simulink model "target_cam_robot_demo"  (Simulink 7.3)
settings: Solver=FixedStepDiscrete  SolverMode=SingleTasking  StartTime=0.0  StopTime=inf  RelTol=1e-3
PreLoadFcn:
  | waijung.modelPreload; % Required for working with Waijung Blockset. Do not remove.
undefined symbols (not defined in the file): A1, A2, A7, B10, B11, B12, C1, C2, C3, C4, C5, G14, H2, H3, H6, H7, HSEOSC, Link, LQFP176, ST, STM32F417IG
libraries: simulink x12, stm32f4_i2c_lib x8, stm32f4_tim_lib x2, stm32f4_io_lib x2, waijung_webserver x2, waijung_socket_lib x2, stm32f4_rcc_lib x1, stm32f4_device_config_lib x1, waijung_addon_module x1
(part 1 of 2)
CloseFcn:
  | waijung.modelClose; % Required for working with Waijung Blockset. Do not remove.
settings Model: Creator=Krisada  LastModifiedBy=Krisada
settings OptimizationCC: OptimizeModelRefInitCode=on  LifeSpan=1
settings HardwareCC: ProdEndianess=LittleEndian  ProdHWDeviceType=ARM Compatible->Cortex - M4  TargetEndianess=LittleEndian  TargetHWDeviceType=ARM Compatible->Cortex - M4
settings RTWCC: SystemTargetFile=stm32f4.tlc  GenerateMakefile=off  TemplateMakefile=ert_default_tmf  Description=STM32F4 Target  ProcessScript=stm32f4_make_rtw_hook
settings CodeAppCC: IgnoreCustomStorageClasses=off
settings STFCustomTargetCC: ModelReferenceCompliant=off  CombineOutputUpdateFcns=on  ERTCustomFileBanners=on  SupportContinuousTime=off  SupportNonInlinedSFcns=off  SystemTargetFile=stm32f4.tlc
settings ERTTargetCC: MultiwordLength=2048  ModelReferenceCompliant=off  ParMdlRefBuildCompliant=off  CompOptLevelCompliant=off  ERTFirstTimeCompliant=off  ModelStepFunctionPrototypeControlCompliant=off  CPPClassGenCompliant=off  ExtModeMexFile=noextcomm  InlinedParameterPlacement=NonHierarchical  ERTSrcFileBannerTemplate=stm32f4_code_template.cgt  ERTHdrFileBannerTemplate=stm32f4_code_template.cgt  ERTDataSrcFileTemplate=stm32f4_code_template.cgt  ERTDataHdrFileTemplate=stm32f4_code_template.cgt  ERTCustomFileTemplate=stm32f4_file_process.tlc

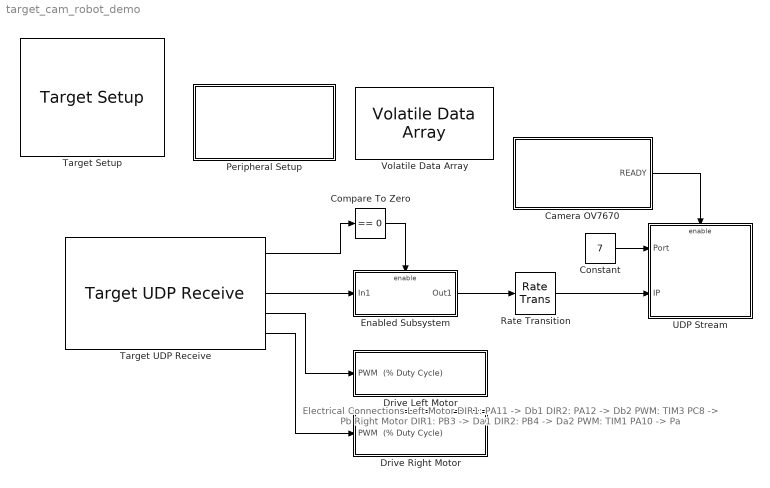
== system target_cam_robot_demo ==
  note: Electrical Connections
      |
      | Left Motor
      | DIR1: PA11 -> Db1
      | DIR2: PA12 ->  Db2
      | PWM: TIM3 PC8 -> Pb
      |
      | Right Motor
      | DIR1: PB3 -> Da1
      | DIR2: PB4 ->  Da2
      | PWM: TIM1 PA10 -> Pa
  Camera OV7670 : Subsystem  mask{camera=OV7670, storagename=ExtRAM, xclkfreq=8MHz(MCO), imgsize=120 x 160, module=1, slvaddr=hex2dec('42'), sampletime=0.01}
      mask prompts: storagename "Output buffer"; xclkfreq "XCLK input frequency"; imgsize "Image size"; module "I2C Module"; slvaddr "I2C Slave address"; sampletime "Sample time (sec)"
      mask init:
      | waijung_image_sensor_callback('init');
      mask StyleString: popup(OV7670),popup(Output|ExtRAM),popup(8MHz(MCO)|24MHz),popup(120 x 160|240 x 320|480 x 640),popup(1|2|3),edit,edit
      mask CallbackString: waijung_image_sensor_callback('camera');|waijung_image_sensor_callback('storagename');|||waijung_image_sensor_callback('module');||
      mask Display: text(0.5, 0.5, '[OV7670]\nPort: I2C1','ver','middle','hor','center');port_label('output', 1,'READY');
  Compare To Zero : simulink/Logic and Bit Operations/Compare To Zero  SystemSampleTime=-1  relop===  LogicOutDataTypeMode=uint8  ZeroCross=off
  Constant : Constant  Value=7  OutDataTypeMode=uint16  OutDataType=fixdt(1, 16)  OutScaling=2^0  OutDataTypeStr=uint16
  Drive Left Motor : Subsystem
  Drive Right Motor : Subsystem
  Enabled Subsystem : Subsystem  TreatAsAtomicUnit=on
  Peripheral Setup : Subsystem
  Rate Transition : RateTransition
  Target Setup : stm32f4_device_config_lib/Target Setup  Priority=100  compiler=GNU ARM  previous_compiler=GNU ARM  mcu=STM32F417IG (LQFP176)  mcustr=STM32F417IG  clockconfig=HSEOSC-8MHz  system_stm32f4xx_c_path=F:\trunk\targets\stm32f4_target\stm32f4\utils\system_stm32f4xx_default\STM32F40_41xxx\hseosc8mhz  showmemoryconfiguration=off  stacksize=0x2000  heapsize=0x2000  enableautocompiledownload=on  fullchiperase=off  programmerinterface=ST-Link  editctrlstr=on  compilercontrolstr=$(patsubst %, -I%, .) -mcpu=cortex-m4 -mthumb -mthumb-interwork -mfloat-abi=hard -mfpu=fpv4-sp-d16 -ffast-math -Wall -Wextra -Ofast  assemblercontrolstr=$(patsubst %, -I%, .) -mcpu=cortex-m4 -mthumb -mthumb-interwork -mfloat-abi=hard -mfpu=fpv4-sp-d16 -ffast-math -Wall -Wextra -Ofast -Wa,-amhls=$(<:.s=.lst) -D__STACK_SIZE=$(STACK_SIZE) -D__HEAP_SIZE=$(HEAP_SIZE)  linkercontrolstr=-T$(LD_SCRIPT) -g -Wl,-Map=$(MAP),--cref,--no-warn-mismatch -mcpu=cortex-m4 -mthumb -mthumb-interwork -mfloat-abi=hard -mfpu=fpv4-sp-d16 -specs=nosys.specs  runafterdownload=on  execprofile=None  profileruart=3  profilerbaud=500000  profilertxpin=D8  profilerinitstr=0.0001,168000000,16800,500000,0  manualsetsampletime=off  sampletime=0.0001  blockid=TargetSetup  systickreloadvalue=16800  hseval=8000000  lastprofileruart=3  hclk=168000000  flashorigin=0x08000000  flashlength=0x100000  ramorigin=0x20000000  ramlength=0x20000  useextram=off
  Target UDP Receive : waijung_socket_lib/Target UDP Receive  conf=TargetReceive  protocol=UDP  port=7  address=192.168.1.21  echo=off  transfer=Non-blocking  timeout=5  datasource=Ports  datatype=uint8  datacount=2  porttype_double=2  porttype_single=0  porttype_int8=0  porttype_uint8=0  porttype_int16=0  porttype_uint16=0  porttype_int32=0  porttype_uint32=0  portpinstr=0  sampletime=inf  blockid=TargetUDPReceive  inputporttype=[]  inputportwidth=[]  inputportlabel={}  outputporttype=[7,5,3,0,0]  outputportwidth=[1,1,4,]  outputportlabel={'Status','Remote Port','Remote IP(1:4)','double D0','double D1'}  compat=0  optionstring="[\"UDP\",\"7\",\"192\",\"168\",\"1\",\"21\",\"Non-blocking\",\"PortData\",\"uint8_t\",\"2\",\"Receive\",\"off\",\"\",\"\",\"\",\"\",\"\",\"\",\"\"]"  options=[7,2,1,5000,0]
  UDP Stream : Subsystem  TreatAsAtomicUnit=on
  Volatile Data Array : waijung_addon_module/Data Storage/Volatile Data Array  conf=Setup  specificaddress=off  storagename=Output  memoryaddress=hex2dec('64000000')  storagetype=uint16  datasize=160*120  varname=VolatileDataArray_Output  datatype=double  datacount=0  portpinstr=0  sampletime=inf  blockid=VolatileDataArray  inputporttype=[]  inputportwidth=[]  inputportlabel={}  outputporttype=[]  outputportwidth=[]  outputportlabel={}  compat=0  optionstring="[\"off\",\"?\",\"Output\",\"uint16\",\"19200\",\"VolatileDataArray_Output\",\"uint16_t\",\"Param1\"]"
  wires:
  Constant/1 -> UDP Stream/1(Port)
  Target UDP Receive/3 -> Enabled Subsystem/1(In1)
  Enabled Subsystem/1(Out1) -> Rate Transition/1
  Target UDP Receive/1 -> Compare To Zero/1
  Compare To Zero/1 -> Enabled Subsystem/Enable
  Camera OV7670/1(READY) -> UDP Stream/Enable
  Rate Transition/1 -> UDP Stream/2(IP)
  Target UDP Receive/4 -> Drive Left Motor/1(PWM  (% Duty Cycle))
  Target UDP Receive/5 -> Drive Right Motor/1(PWM  (% Duty Cycle))

== system target_cam_robot_demo/Camera OV7670 ==
  Capture_ : Subsystem  TreatAsAtomicUnit=on
  Init_ : Subsystem
  Logical Operator : Logic  Operator=NOT  AllPortsSameDT=off  OutDataTypeMode=boolean  LogicDataType=fixdt(0, 8)  OutDataTypeStr=boolean
  Memory : Memory  InheritSampleTime=on
  Rate Transition : RateTransition  OutPortSampleTime=sampletime
  READY : Outport  OutDataType=fixdt(1, 16)  OutScaling=2^0
  wires:
  Rate Transition/1 -> Capture_/Enable
  Logical Operator/1 -> Init_/Enable
  Memory/1 -> Rate Transition/1, Logical Operator/1
  Init_/1(Out1) -> Memory/1
  Capture_/1(SUCCESS) -> READY/1

== system target_cam_robot_demo/Drive Left Motor ==
  PWM  (% Duty Cycle) : Inport
  Abs : Abs  OutDataType=fixdt(1, 16)  OutScaling=2^0
  Basic PWM : S-Function  FunctionName=stm32f4_basicpwm  Parameters=timer,pwmperiod,ch1pin,ch2pin,ch3pin,ch4pin,sampletime,sampletimestr,blockid,apb,portstr,pinstr,pinmat,timarr,timprescale,chmat,polaritystr  EnableBusSupport=off  mask(stm32f4_basicpwm){timer=3, pwmperiod=0.005, polarity=Active High, polaritystr=TIM_OCPolarity_High, ch1pin=Not available - Do not use, ch2pin=Not available - Do not use, ch3pin=C8, ch4pin=Not available - Do not use, sampletime=-1, sampletimestr=0.0001, blockid=DriveLeftMotorBasicPWM, portpinstr=,,C8,, enablecustomportlabel=off, cinputportlabel=In1, In2, In3, In4, coutputportlabel=0, apb=1, portstr=["C"], pinstr=["GPIO_Pin_8"], pinmat=[1 8], timarr=59999, timprescale=6, chmat=[3]}
      mask prompts: pwmperiod "PWM Period (seconds)"; ch1pin "Channel 1"; ch2pin "Channel 2"; ch3pin "Channel 3"; ch4pin "Channel 4"; sampletime "Sample time (sec)"; sampletimestr "Compiled sample time (sec) in string"; portpinstr "Port pin string"; enablecustomportlabel "Enable custom port labels"; cinputportlabel "Custom input port labels (Ex. In1, In2, In3)"; coutputportlabel "Custom output port labels (Ex. Out1, Out2, Out3)"; portstr "Port string"; pinstr "Pin string"; pinmat "Pin matrix"; timarr "Timer ARR"; timprescale "Timer PRESCALE"; chmat "Channel order"
      mask help:
      | This block implements basic Edge-aligned Pulse Width Modulation (PWM) generation.
      | All timers are 16-bit. The PWM period is fixed (per timer).
      mask init:
      | stm32f4_basicpwm_callback('init');
      mask Help: web(fullfile(waijungdocroot,'stm32f4_basicpwm.htm'),'-browser')
      mask StyleString: popup(1|2|3|4|5|8|9|10|11|12|13|14),edit,popup(Active High|Active Low),edit,popup(Not available - Do not use|A6|C6|B4),popup(Not available - Do not use|A7|C7|B5),popup(Not available - Do not use|B0|C8),popup(Not available - Do not use|B1|C9),edit,edit,edit,edit,checkbox,edit,edit,edit,edit,edit,edit,edit,edit,edit
      mask CallbackString: stm32f4_basicpwm_callback('timer');|stm32f4_basicpwm_callback('pwmperiod');|stm32f4_basicpwm_callback('polarity');||stm32f4_basicpwm_callback('ch1pin');|stm32f4_basicpwm_callback('ch2pin');|stm32f4_basicpwm_callback('ch3pin');|stm32f4_basicpwm_callback('ch4pin');|stm32f4_basicpwm_callback('sampletime');|stm32f4_basicpwm_callback('sampletimestr');|stm32f4_basicpwm_callback('blockid');||stm32f4_basicpwm_callback('enablecustomportlabel');|||||||||
      mask Display: text(0.95, 0.5, 'Timer: 3\nPolarity: Active High\nPeriod (sec) 0.005\nTs (sec): 0.0001','ver','middle','hor','right');port_label('input', 1,'CH3 (C8)')
  CCW : Subsystem  TreatAsAtomicUnit=on
  CW : Subsystem  TreatAsAtomicUnit=on
  Demux : Demux  Outputs=2
  Digital Output : stm32f4_io_lib/Digital Output  use_bitband=on  port=A  speed=100  porttype=Open Drain  porttypestr=OD  use_pin0=off  use_pin1=off  use_pin2=off  use_pin3=off  use_pin4=off  use_pin5=off  use_pin6=off  use_pin7=off  use_pin8=off  use_pin9=off  use_pin10=off  use_pin11=on  use_pin12=on  use_pin13=off  use_pin14=off  use_pin15=off  pinstr=GPIO_Pin_11 | GPIO_Pin_12  usedpinarray="[0  0  0  0  0  0  0  0  0  0  0  1  1  0  0  0]"  bitbandingstr=|  sampletime=-1  sampletimestr=0.0001  blockid=DriveLeftMotorDigitalOutput  enablecustomportlabel=off  globalinit=off  cinputportlabel=In1, In2  coutputportlabel=0
      | #define DriveLeftMotorDigitalOutput_A11 Peripheral_BB(GPIOA->ODR, 11)  /* Output pin */
      | #define DriveLeftMotorDigitalOutput_A12 Peripheral_BB(GPIOA->ODR, 12)  /* Output pin */
  If : If  ElseIfExpressions=u1<0
  Merge : Merge  Inputs=3  InitialOutput=[0 0]
  STOP : Subsystem  TreatAsAtomicUnit=on
  wires:
  Abs/1 -> Basic PWM/1
  If/1 -> CW/Action
  If/2 -> CCW/Action
  If/3 -> STOP/Action
  CW/1(DIR) -> Merge/1
  CCW/1(DIR) -> Merge/2
  STOP/1(DIR) -> Merge/3
  Merge/1 -> Demux/1
  Demux/1 -> Digital Output/1
  PWM  (% Duty Cycle)/1 -> Abs/1, If/1
  Demux/2 -> Digital Output/2

== system target_cam_robot_demo/Drive Right Motor ==
  PWM  (% Duty Cycle) : Inport
  Abs : Abs  OutDataType=fixdt(1, 16)  OutScaling=2^0
  Basic PWM : S-Function  FunctionName=stm32f4_basicpwm  Parameters=timer,pwmperiod,ch1pin,ch2pin,ch3pin,ch4pin,sampletime,sampletimestr,blockid,apb,portstr,pinstr,pinmat,timarr,timprescale,chmat,polaritystr  EnableBusSupport=off  mask(stm32f4_basicpwm){timer=1, pwmperiod=0.005, polarity=Active High, polaritystr=TIM_OCPolarity_High, ch1pin=Not available - Do not use, ch2pin=Not available - Do not use, ch3pin=A10, ch4pin=Not available - Do not use, sampletime=-1, sampletimestr=0.0001, blockid=DriveRightMotorBasicPWM, portpinstr=,,A10,, enablecustomportlabel=off, cinputportlabel=In1, In2, In3, In4, coutputportlabel=0, apb=2, portstr=["A"], pinstr=["GPIO_Pin_10"], pinmat=[1 10], timarr=64614, timprescale=12, chmat=[3]}
      mask prompts: pwmperiod "PWM Period (seconds)"; ch1pin "Channel 1"; ch2pin "Channel 2"; ch3pin "Channel 3"; ch4pin "Channel 4"; sampletime "Sample time (sec)"; sampletimestr "Compiled sample time (sec) in string"; portpinstr "Port pin string"; enablecustomportlabel "Enable custom port labels"; cinputportlabel "Custom input port labels (Ex. In1, In2, In3)"; coutputportlabel "Custom output port labels (Ex. Out1, Out2, Out3)"; portstr "Port string"; pinstr "Pin string"; pinmat "Pin matrix"; timarr "Timer ARR"; timprescale "Timer PRESCALE"; chmat "Channel order"
      mask help:
      | This block implements basic Edge-aligned Pulse Width Modulation (PWM) generation.
      | All timers are 16-bit. The PWM period is fixed (per timer).
      mask init:
      | stm32f4_basicpwm_callback('init');
      mask Help: web(fullfile(waijungdocroot,'stm32f4_basicpwm.htm'),'-browser')
      mask StyleString: popup(1|2|3|4|5|8|9|10|11|12|13|14),edit,popup(Active High|Active Low),edit,popup(Not available - Do not use|E9|A8),popup(Not available - Do not use|E11|A9),popup(Not available - Do not use|E13|A10),popup(Not available - Do not use|E14|A11),edit,edit,edit,edit,checkbox,edit,edit,edit,edit,edit,edit,edit,edit,edit
      mask CallbackString: stm32f4_basicpwm_callback('timer');|stm32f4_basicpwm_callback('pwmperiod');|stm32f4_basicpwm_callback('polarity');||stm32f4_basicpwm_callback('ch1pin');|stm32f4_basicpwm_callback('ch2pin');|stm32f4_basicpwm_callback('ch3pin');|stm32f4_basicpwm_callback('ch4pin');|stm32f4_basicpwm_callback('sampletime');|stm32f4_basicpwm_callback('sampletimestr');|stm32f4_basicpwm_callback('blockid');||stm32f4_basicpwm_callback('enablecustomportlabel');|||||||||
      mask Display: text(0.95, 0.5, 'Timer: 1\nPolarity: Active High\nPeriod (sec) 0.005\nTs (sec): 0.0001','ver','middle','hor','right');port_label('input', 1,'CH3 (A10)')
  CCW : Subsystem  TreatAsAtomicUnit=on
  CW : Subsystem  TreatAsAtomicUnit=on
  Demux : Demux  Outputs=2
  Digital Output : stm32f4_io_lib/Digital Output  use_bitband=on  port=B  speed=100  porttype=Open Drain  porttypestr=OD  use_pin0=off  use_pin1=off  use_pin2=off  use_pin3=on  use_pin4=on  use_pin5=off  use_pin6=off  use_pin7=off  use_pin8=off  use_pin9=off  use_pin10=off  use_pin11=off  use_pin12=off  use_pin13=off  use_pin14=off  use_pin15=off  pinstr=GPIO_Pin_3 | GPIO_Pin_4  usedpinarray="[0  0  0  1  1  0  0  0  0  0  0  0  0  0  0  0]"  bitbandingstr=|  sampletime=-1  sampletimestr=0.0001  blockid=DriveRightMotorDigitalOutput  enablecustomportlabel=off  globalinit=off  cinputportlabel=In1, In2  coutputportlabel=0
      | #define DriveRightMotorDigitalOutput_B3 Peripheral_BB(GPIOB->ODR, 3)  /* Output pin */
      | #define DriveRightMotorDigitalOutput_B4 Peripheral_BB(GPIOB->ODR, 4)  /* Output pin */
  If : If  ElseIfExpressions=u1<0
  Merge : Merge  Inputs=3  InitialOutput=[0 0]
  STOP : Subsystem  TreatAsAtomicUnit=on
  wires:
  PWM  (% Duty Cycle)/1 -> If/1, Abs/1
  Demux/2 -> Digital Output/2
  Demux/1 -> Digital Output/1
  Merge/1 -> Demux/1
  STOP/1(DIR) -> Merge/3
  CCW/1(DIR) -> Merge/2
  CW/1(DIR) -> Merge/1
  If/3 -> STOP/Action
  If/2 -> CCW/Action
  If/1 -> CW/Action
  Abs/1 -> Basic PWM/1

== system target_cam_robot_demo/Enabled Subsystem ==
  In1 : Inport  OutDataType=fixdt(1, 16)  OutScaling=2^0
  Enable : EnablePort
  Out1 : Outport  OutDataType=fixdt(1, 16)  OutScaling=2^0  InitialOutput=[192 168 1 48]
  wires:
  In1/1 -> Out1/1

== system target_cam_robot_demo/Peripheral Setup ==
  Ethernet Application Setup : waijung_webserver/Ethernet Application Setup  conf=Setup  ipaddress=192.168.1.31  netmask=255.255.255.0  gateway=192.168.1.1  macaddress=02-00-00-00-00-00  dhcp=off  timerscaler=100  portpinstr=0  sampletime=0.0001  blockid=PeripheralSetupEthernetApplicationSetup  inputporttype=[]  inputportwidth=[]  inputportlabel={}  outputporttype=[]  outputportwidth=[]  outputportlabel={}  compat=0  optionstring="[\"Dummy\",\"192\",\"168\",\"1\",\"31\",\"255\",\"255\",\"255\",\"0\",\"192\",\"168\",\"1\",\"1\",\"02\",\"00\",\"00\",\"00\",\"00\",\"00\",\"off\",\"100\"]"
  Ethernet Link Setup : waijung_webserver/Ethernet Link Setup  conf=Setup  interfacepin=Profile #2  wj_interfacetype=MII  pin_mdio=A2  pin_mdc=C1  pin_pps=Not used  pin_crs=H2  pin_col=H3  pin_dv=A7  pin_rxclk=A1  pin_rxer=B10  pin_rxd0=C4  pin_rxd1=C5  pin_rxd2=H6  pin_rxd3=H7  pin_txclk=C3  pin_txen=B11  pin_txd0=B12  pin_txd1=G14  pin_txd2=C2  pin_txd3=E2  portpinstr=H2,A1,A2,H3,A7,H6,H7,E2,B10,B11,B12,G14,C1,C2,C3,C4,C5  sampletime=inf  blockid=PeripheralSetupEthernetLinkSetup  inputporttype=[]  inputportwidth=[]  inputportlabel={}  outputporttype=[]  outputportwidth=[]  outputportlabel={}  compat=0  optionstring="[\"xxx\",\"on\",\"on\",\"on\",\"off\",\"on\",\"off\",\"on\",\"on\",\"off\",\"on\",\"on\",\"on\",\"on\",\"on\",\"on\",\"on\",\"off\",\"on\",\"on\",\"on\",\"on\",\"on\",\"on\",\"on\",\"on\",\"on\",\"on\",\"H\",\"2\",\"A\",\"1\",\"A\",\"2\",\"H\",\"3\",\"A\",\"7\",\"H\",\"6\",\"H\",\"7\",\"N\",\"ot used\",\"E\",\"2\",\"B\",\"10\",\"B\",\"11\",\"B\",\"12\",\"G\",\"14\",\"C\",\"1\",\"C\",\"2\",\"C\",\"3\",\"C\",\"4\",\"C\",\"5\",\"MII\"]"
  I2C Master Setup : S-Function  FunctionName=stm32f4_i2c  Parameters=configuration,module,transfer,clkspeed,timeout,sdapin,sclpin,writecount,readcount,inputtypearray,outputtypearray,confstr,sampletime,sampletimestr,blockid  EnableBusSupport=off  mask(stm32f4_i2c){configuration=Setup, module=1, lastmodule=1, transfer=Blocking, dutycycle=TLow/THigh = 2, clkspeed=100, timeout=25, writecount=0, readcount=0, sdapin=B7, sclpin=B6, waitwritetime=0, inputtypearray=[0], outputtypearray=[0], confstr=["B","7","B","6","1","1","6","0","I2C_DutyCycle_2","0","off"], sampletime=-1, sampletimestr=0.0001, blockid=PeripheralSetupI2CMasterSetup}
      mask prompts: module "I2C Module"; lastmodule "Last module"; transfer "Transfer mode"; dutycycle "Duty cycle in fast mode"; clkspeed "Clock speed (kHz)"; timeout "Timeout (ms)"; writecount "Bytes write count"; readcount "Bytes read count"; sdapin "SDA pin"; sclpin "SCL pin"; waitwritetime "Wait write time (ms), default is 0"; inputtypearray "Input type array"; outputtypearray "Output type array"; confstr "Configuration string"; sampletime "Sample time (sec)"; sampletimestr "Compiled sample time (sec) in string"
      mask init:
      | stm32f4_i2c_callback('init');
      mask Help: web(fullfile(waijungdocroot,'stm32f4_i2c_setup.htm'), '-browser')
      mask StyleString: popup(Setup|Transaction),popup(1|2|3),edit,popup(Blocking|Non-blocking),popup(TLow/THigh = 16/9|TLow/THigh = 2),edit,edit,edit,edit,popup(Not used|B7|B9),popup(Not used|B6|B8),edit,edit,edit,edit,edit,edit,edit
      mask CallbackString: stm32f4_i2c_callback('configuration');|stm32f4_i2c_callback('module');|||stm32f4_i2c_callback('dutycycle');|||stm32f4_i2c_callback('writecount');|stm32f4_i2c_callback('readcount');|stm32f4_i2c_callback('sdapin');|stm32f4_i2c_callback('sclpin');||||stm32f4_i2c_callback('confstr');|stm32f4_i2c_callback('sampletime');|stm32f4_i2c_callback('sampletimestr');|stm32f4_i2c_callback('blockid');
      mask Display: text(0.5, 0.5, 'Module: I2C1\nClock: 100kHz\nSDA/SCL Pin: B7/B6','ver','middle','hor','center');
  MCO : stm32f4_rcc_lib/MCO  conf=MCO  module=1  source=HSE  div=Div_1  sampletime=inf  sampletimestr=0.0001  blockid=PeripheralSetupMCO  inputarray=[]  inputlabelarray={}  outputarray=[]  outputlabelarray={}  compat=0  confstr="[\"1\",\"HSE\",\"Div_1\"]"

== system target_cam_robot_demo/UDP Stream ==
  Port : Inport  OutDataType=fixdt(1, 16)  OutScaling=2^0
  IP : Inport  Port=2  OutDataType=fixdt(1, 16)  OutScaling=2^0
  Enable : EnablePort
  Target UDP Send : waijung_socket_lib/Target UDP Send  conf=TargetSend  protocol=UDP  variableipport=on  port=7  address=192.168.1.33  echo=off  transfer=Non-blocking  timeout=5  datasource=BufferStream  streamsource=Output  streamsize=1024  datatype=uint16  datacount=120*160  porttype_double=0  porttype_single=0  porttype_int8=0  porttype_uint8=0  porttype_int16=0  porttype_uint16=0  porttype_int32=0  porttype_uint32=1  portpinstr=0  sampletime=-1  blockid=UDPStreamTargetUDPSend  inputporttype=[5,3,]  inputportwidth=[1,4,]  inputportlabel={'Port','IP',}  outputporttype=[7]  outputportwidth=[]  outputportlabel={'Status'}  compat=0  optionstring="[\"UDP\",\"7\",\"192\",\"168\",\"1\",\"33\",\"Non-blocking\",\"BufferStream\",\"uint16_t\",\"120*160\",\"Send\",\"off\",\"on\",\"Output\",\"VolatileDataArray_Output\",\"uint16\",\"19200\",\"38400\",\"1024\"]"  options=[7,2,0,5000,1]
  Terminator : Terminator
  wires:
  Port/1 -> Target UDP Send/1
  IP/1 -> Target UDP Send/2
  Target UDP Send/1 -> Terminator/1

== system target_cam_robot_demo/Camera OV7670/Capture_ ==
  Enable : EnablePort
  Compare To Zero : simulink/Logic and Bit Operations/Compare To Zero  SystemSampleTime=-1  relop===  LogicOutDataTypeMode=uint8  ZeroCross=off
  DCMI Capture : S-Function  FunctionName=stm32f4_dcmi  Parameters=conf,inputporttype,inputportwidth,outputporttype,outputportwidth,optionstring,sampletime,blockid  EnableBusSupport=off  mask(stm32f4_dcmi){conf=DCMI, capturemode=SnapShot, synchronizemode=Hardware, pclkpolarity=Falling, vspolarity=High, hspolarity=High, capturerate=All, capturesize=120*160*2, storagename=<Manual Configure>, varname=VolatileDataArray_Output, storagetype=uint16, storagesize=120*160, remap=Profile #2, sampletime=inf, blockid=CameraOV7670Capture_DCMICapture, inputporttype=[], inputportwidth=[], inputportlabel={}, outputporttype=[7], outputportwidth=[], outputportlabel={'Status'}, compat=0, optionstring=["DCMI","SnapShot","Hardware","Falling","High","High","All","0","HalfWord","9600","0","0","VolatileDataArray_Output"," "," "," ","1","0","0","0","0","0","0","1","1","A","6","I","5","H","8","H","9","H","10","H","11","H","12","H","14","I","4","I","6","I","7"], portpinstr=A6,I5,H8,H9,H10,H11,H12,H14,I4,I6,I7}
      mask prompts: conf "Configuration"; capturemode "Capture mode"; synchronizemode "Synchronization Mode"; pclkpolarity "Pixel clock polarity"; vspolarity "Vertical synchronization polarity"; hspolarity "Horizontal synchronization polarity"; capturerate "Capture rate"; capturesize "Capture data size (Bytes)"; storagename "Output buffer"; varname "Output buffer var name"; storagetype "Output buffer var type"; storagesize "Output buffer size (Total bytes must be equal to, or greater than DMA Transfer size)"; remap "Remap DCMI pins"; sampletime "Sample time (sec)"; inputporttype "Input port"; inputportwidth "Input Port Width"; inputportlabel "Input port label"; outputporttype "Output port"; outputportwidth "Output Port Width"; outputportlabel "Output port label"; compat "Compatibility (Reserved for future use)"; optionstring "Configuration String"; portpinstr "Port Pin String"
      mask help:
      | Synchronize mode:
      |  - Hardware: Hardware synchronization data capture is synchronized with the HSYNC/VSYNC signals.
      |  - Embedded: Embedded synchronization data capture is synchronized with synchronization codes embedded in the data flow.
      | Pixel clock polarity:
      |  - Falling: Pixel clock active on Falling edge.
      |  - Rising: Pixel clock active on Rising edge.
      | Vertical, Horizontal sychronization polarity:
      |  - Low: vertical synchronization active Low.
      |  - High: Vertical synchronization active High.
      | Capture rate:
      |  - All: All frames are captured.
      |  - 1of2: Every alternate frame captured.
      |  - 1of4: On frame in 4 frames captured.
      | Pins Profile:
      | Set of configuration pins for: PIXCLK, VSYNC, HSYNC, D0, D1, .., D7 corresponding.
      |  - Profile #1: PA6, PB7, PA4, PC6, PC7,  PE0,  PE1,  PE4,  PB6, PE5, PE6
      |  - Profile #2: PA6, PI5, PH8, PH9, PH10, PH11, PH12, PH14, PI4, PI6, PI7
      mask init:
      | stm32f4_dcmi_callback('init');
      mask Help: web(fullfile(waijungdocroot,'stm32f4_dcmi.htm'), '-browser')
      mask StyleString: popup(DCMI),popup(Continuous|SnapShot),popup(Hardware|Embedded),popup(Falling|Rising),popup(High|Low),popup(High|Low),popup(All|1of2|1of4),edit,popup(<Manual Configure>),edit,popup(double|single|int8|uint8|int16|uint16|int32|uint32),edit,popup(Profile #1|Profile #2),edit,edit,edit,edit,edit,edit,edit,edit,edit,edit,edit
      mask CallbackString: stm32f4_dcmi_callback('conf');||||||||stm32f4_dcmi_callback('storagename');|||stm32f4_dcmi_callback('storagesize');|stm32f4_dcmi_callback('remap');|stm32f4_dcmi_callback('sampletime');|stm32f4_dcmi_callback('blockid');|||||||||
      mask Display: text(0.05, 0.5, 'Size: 38400\nPins: Profile #2\nTs (sec): 0.01','ver','middle','hor','left'); port_label('output', 1,'Status');
  SUCCESS : Outport  OutDataType=fixdt(1, 16)  OutScaling=2^0
  wires:
  DCMI Capture/1 -> Compare To Zero/1
  Compare To Zero/1 -> SUCCESS/1

== system target_cam_robot_demo/Camera OV7670/Init_ ==
  Enable : EnablePort
  While Iterator_ : Subsystem  TreatAsAtomicUnit=on
  Out1 : Outport
  wires:
  While Iterator_/1(Ready) -> Out1/1

== system target_cam_robot_demo/Drive Left Motor/CCW ==
  Action Port : ActionPort  ActionType=elseif
  Constant : Constant  Value=0  OutDataType=fixdt(1, 16)  OutScaling=2^0
  Constant1 : Constant  OutDataType=fixdt(1, 16)  OutScaling=2^0
  Mux : Mux  Inputs=2
  DIR : Outport  OutDataType=fixdt(1, 16)  OutScaling=2^0  InitialOutput=[0 0]
  wires:
  Mux/1 -> DIR/1
  Constant1/1 -> Mux/2
  Constant/1 -> Mux/1

== system target_cam_robot_demo/Drive Left Motor/CW ==
  Action Port : ActionPort  ActionType=then
  Constant : Constant  OutDataType=fixdt(1, 16)  OutScaling=2^0
  Constant1 : Constant  Value=0  OutDataType=fixdt(1, 16)  OutScaling=2^0
  Mux : Mux  Inputs=2
  DIR : Outport  OutDataType=fixdt(1, 16)  OutScaling=2^0  InitialOutput=[0 0]
  wires:
  Constant/1 -> Mux/1
  Constant1/1 -> Mux/2
  Mux/1 -> DIR/1

== system target_cam_robot_demo/Drive Left Motor/STOP ==
  Action Port : ActionPort  ActionType=else
  Constant : Constant  Value=0  OutDataType=fixdt(1, 16)  OutScaling=2^0
  Constant1 : Constant  Value=0  OutDataType=fixdt(1, 16)  OutScaling=2^0
  Mux : Mux  Inputs=2
  DIR : Outport  OutDataType=fixdt(1, 16)  OutScaling=2^0  InitialOutput=[0 0]
  wires:
  Constant/1 -> Mux/1
  Constant1/1 -> Mux/2
  Mux/1 -> DIR/1

== system target_cam_robot_demo/Drive Right Motor/CCW ==
  Action Port : ActionPort  ActionType=elseif
  Constant : Constant  Value=0  OutDataType=fixdt(1, 16)  OutScaling=2^0
  Constant1 : Constant  OutDataType=fixdt(1, 16)  OutScaling=2^0
  Mux : Mux  Inputs=2
  DIR : Outport  OutDataType=fixdt(1, 16)  OutScaling=2^0  InitialOutput=[0 0]
  wires:
  Constant/1 -> Mux/1
  Constant1/1 -> Mux/2
  Mux/1 -> DIR/1

== system target_cam_robot_demo/Drive Right Motor/CW ==
  Action Port : ActionPort  ActionType=then
  Constant : Constant  OutDataType=fixdt(1, 16)  OutScaling=2^0
  Constant1 : Constant  Value=0  OutDataType=fixdt(1, 16)  OutScaling=2^0
  Mux : Mux  Inputs=2
  DIR : Outport  OutDataType=fixdt(1, 16)  OutScaling=2^0  InitialOutput=[0 0]
  wires:
  Mux/1 -> DIR/1
  Constant1/1 -> Mux/2
  Constant/1 -> Mux/1

== system target_cam_robot_demo/Drive Right Motor/STOP ==
  Action Port : ActionPort  ActionType=else
  Constant : Constant  Value=0  OutDataType=fixdt(1, 16)  OutScaling=2^0
  Constant1 : Constant  Value=0  OutDataType=fixdt(1, 16)  OutScaling=2^0
  Mux : Mux  Inputs=2
  DIR : Outport  OutDataType=fixdt(1, 16)  OutScaling=2^0  InitialOutput=[0 0]
  wires:
  Mux/1 -> DIR/1
  Constant1/1 -> Mux/2
  Constant/1 -> Mux/1

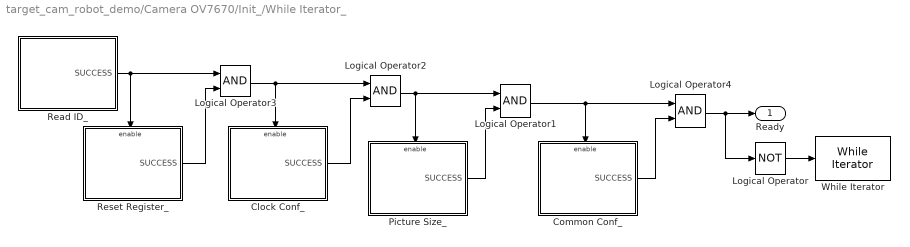
== system target_cam_robot_demo/Camera OV7670/Init_/While Iterator_ ==
  Clock Conf_ : Subsystem
  Common Conf_ : Subsystem
  Logical Operator : Logic  Operator=NOT  AllPortsSameDT=off  OutDataTypeMode=boolean  LogicDataType=fixdt(0, 8)  OutDataTypeStr=boolean
  Logical Operator{1..4} (4 alike) : Logic  AllPortsSameDT=off  OutDataTypeMode=boolean  LogicDataType=fixdt(0, 8)  OutDataTypeStr=boolean
  Picture Size_ : Subsystem
  Read ID_ : Subsystem
  Reset Register_ : Subsystem
  While Iterator : WhileIterator  MaxIters=-1  WhileBlockType=do-while
  Ready : Outport  OutDataType=fixdt(1, 16)  OutScaling=2^0
  wires:
  Common Conf_/1(SUCCESS) -> Logical Operator4/2
  Logical Operator4/1 -> Ready/1, Logical Operator/1
  Logical Operator2/1 -> Picture Size_/Enable, Logical Operator1/1
  Clock Conf_/1(SUCCESS) -> Logical Operator2/2
  Reset Register_/1(SUCCESS) -> Logical Operator3/2
  Logical Operator/1 -> While Iterator/1
  Logical Operator1/1 -> Logical Operator4/1, Common Conf_/Enable
  Picture Size_/1(SUCCESS) -> Logical Operator1/2
  Read ID_/1(SUCCESS) -> Logical Operator3/1, Reset Register_/Enable
  Logical Operator3/1 -> Logical Operator2/1, Clock Conf_/Enable

== system target_cam_robot_demo/Camera OV7670/Init_/While Iterator_/Clock Conf_ ==
  Enable : EnablePort
  Logical Operator : Logic  Operator=NOT  AllPortsSameDT=off  OutDataTypeMode=boolean  LogicDataType=fixdt(0, 8)  OutDataTypeStr=boolean
  Memory : Memory  InheritSampleTime=on
  Subsystem : Subsystem
  SUCCESS : Outport  OutDataType=fixdt(1, 16)  OutScaling=2^0
  wires:
  Subsystem/1(Out1) -> SUCCESS/1, Memory/1
  Logical Operator/1 -> Subsystem/Enable
  Memory/1 -> Logical Operator/1

== system target_cam_robot_demo/Camera OV7670/Init_/While Iterator_/Common Conf_ ==
  Enable : EnablePort
  Logical Operator : Logic  Operator=NOT  AllPortsSameDT=off  OutDataTypeMode=boolean  LogicDataType=fixdt(0, 8)  OutDataTypeStr=boolean
  Memory : Memory  InheritSampleTime=on
  Subsystem : Subsystem
  SUCCESS : Outport  OutDataType=fixdt(1, 16)  OutScaling=2^0
  wires:
  Subsystem/1(Out1) -> SUCCESS/1, Memory/1
  Logical Operator/1 -> Subsystem/Enable
  Memory/1 -> Logical Operator/1

== system target_cam_robot_demo/Camera OV7670/Init_/While Iterator_/Picture Size_ ==
  Enable : EnablePort
  Logical Operator : Logic  Operator=NOT  AllPortsSameDT=off  OutDataTypeMode=boolean  LogicDataType=fixdt(0, 8)  OutDataTypeStr=boolean
  Memory : Memory  InheritSampleTime=on
  Subsystem : Subsystem
  SUCCESS : Outport  OutDataType=fixdt(1, 16)  OutScaling=2^0
  wires:
  Memory/1 -> Logical Operator/1
  Logical Operator/1 -> Subsystem/Enable
  Subsystem/1(Out1) -> Memory/1, SUCCESS/1

== system target_cam_robot_demo/Camera OV7670/Init_/While Iterator_/Read ID_ ==
  Logical Operator : Logic  Operator=NOT  AllPortsSameDT=off  OutDataTypeMode=boolean  LogicDataType=fixdt(0, 8)  OutDataTypeStr=boolean
  Memory : Memory  InheritSampleTime=on
  Subsystem_ : Subsystem
  SUCCESS : Outport  OutDataType=fixdt(1, 16)  OutScaling=2^0
  wires:
  Memory/1 -> Logical Operator/1
  Logical Operator/1 -> Subsystem_/Enable
  Subsystem_/1(Out1) -> Memory/1, SUCCESS/1

== system target_cam_robot_demo/Camera OV7670/Init_/While Iterator_/Reset Register_ ==
  Enable : EnablePort
  Logical Operator : Logic  Operator=NOT  AllPortsSameDT=off  OutDataTypeMode=boolean  LogicDataType=fixdt(0, 8)  OutDataTypeStr=boolean
  Memory : Memory  InheritSampleTime=on
  Subsystem : Subsystem
  SUCCESS : Outport  OutDataType=fixdt(1, 16)  OutScaling=2^0
  wires:
  Subsystem/1(Out1) -> SUCCESS/1, Memory/1
  Logical Operator/1 -> Subsystem/Enable
  Memory/1 -> Logical Operator/1

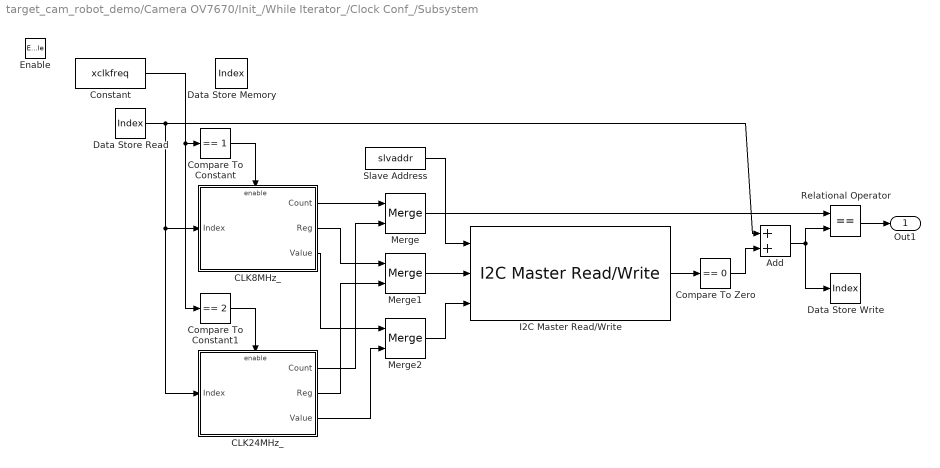
== system target_cam_robot_demo/Camera OV7670/Init_/While Iterator_/Clock Conf_/Subsystem ==
  Enable : EnablePort
  Add : Sum  OutDataType=fixdt(1, 16)  OutScaling=2^-10
  CLK24MHz_ : Subsystem  TreatAsAtomicUnit=on
  CLK8MHz_ : Subsystem  TreatAsAtomicUnit=on
  Compare To Constant : simulink/Logic and Bit Operations/Compare To Constant  SystemSampleTime=-1  relop===  const=1  LogicOutDataTypeMode=boolean  ZeroCross=off
  Compare To Constant1 : simulink/Logic and Bit Operations/Compare To Constant  SystemSampleTime=-1  relop===  const=2  LogicOutDataTypeMode=boolean  ZeroCross=off
  Compare To Zero : simulink/Logic and Bit Operations/Compare To Zero  SystemSampleTime=-1  relop===  LogicOutDataTypeMode=uint8  ZeroCross=off
  Constant : Constant  Value=xclkfreq  OutDataType=fixdt(1, 16)  OutScaling=2^0
  Data Store Memory : DataStoreMemory  DataStoreName=Index  ReadBeforeWriteMsg=warning  WriteAfterWriteMsg=warning  WriteAfterReadMsg=warning  DataType=uint8  OutDataType=fixdt(1, 16)  OutScaling=2^0  OutDataTypeStr=uint8
  Data Store Read : DataStoreRead  DataStoreName=Index  SampleTime=-1
  Data Store Write : DataStoreWrite  DataStoreName=Index  SampleTime=-1
  I2C Master Read/Write : stm32f4_i2c_lib/I2C Master Read//Write  configuration=Transaction  module=1  lastmodule=3  transfer=Blocking  dutycycle=TLow/THigh = 2  clkspeed=400  timeout=25  writecount=2  readcount=0  sdapin=C9  sclpin=A8  waitwritetime=5  forcestop=off  inputtypearray=[3 3 3 3]  outputtypearray=[1 3]  confstr="[\"C\",\"9\",\"A\",\"8\",\"1\",\"1\",\"6\",\"0\",\"I2C_DutyCycle_2\",\"5\",\"off\"]"  sampletime=-1  sampletimestr=-1  blockid=CameraOV7670Init_WhileIterator_ClockConf_SubsystemI2CMasterReadWrite
  Merge : Merge
  Merge1 : Merge
  Merge2 : Merge
  Relational Operator : RelationalOperator  Operator===  LogicOutDataTypeMode=boolean  LogicDataType=fixdt(0, 8)  OutDataTypeStr=boolean
  Slave Address : Constant  Value=slvaddr  OutDataTypeMode=uint8  OutDataType=fixdt(1, 16)  OutScaling=2^0  OutDataTypeStr=uint8
  Out1 : Outport
  wires:
  Merge2/1 -> I2C Master Read/Write/3
  Merge1/1 -> I2C Master Read/Write/2
  Merge/1 -> Relational Operator/1
  Constant/1 -> Compare To Constant1/1, Compare To Constant/1
  CLK24MHz_/3(Value) -> Merge2/2
  CLK24MHz_/2(Reg) -> Merge1/2
  CLK24MHz_/1(Count) -> Merge/2
  CLK8MHz_/3(Value) -> Merge2/1
  CLK8MHz_/2(Reg) -> Merge1/1
  CLK8MHz_/1(Count) -> Merge/1
  Compare To Constant1/1 -> CLK24MHz_/Enable
  Compare To Constant/1 -> CLK8MHz_/Enable
  Slave Address/1 -> I2C Master Read/Write/1
  Data Store Read/1 -> CLK24MHz_/1(Index), CLK8MHz_/1(Index), Add/1
  I2C Master Read/Write/1 -> Compare To Zero/1
  Compare To Zero/1 -> Add/2
  Add/1 -> Relational Operator/2, Data Store Write/1
  Relational Operator/1 -> Out1/1

== system target_cam_robot_demo/Camera OV7670/Init_/While Iterator_/Common Conf_/Subsystem ==
  Enable : EnablePort
  Add : Sum  OutDataType=fixdt(1, 16)  OutScaling=2^-10
  Compare To Zero : simulink/Logic and Bit Operations/Compare To Zero  SystemSampleTime=-1  relop===  LogicOutDataTypeMode=uint8  ZeroCross=off
  Data Store Memory : DataStoreMemory  DataStoreName=Index  ReadBeforeWriteMsg=warning  WriteAfterWriteMsg=warning  WriteAfterReadMsg=warning  DataType=uint8  OutDataType=fixdt(1, 16)  OutScaling=2^0  OutDataTypeStr=uint8
  Data Store Read : DataStoreRead  DataStoreName=Index  SampleTime=-1
  Data Store Write : DataStoreWrite  DataStoreName=Index  SampleTime=-1
  I2C Master Read/Write : stm32f4_i2c_lib/I2C Master Read//Write  configuration=Transaction  module=1  lastmodule=3  transfer=Blocking  dutycycle=TLow/THigh = 2  clkspeed=400  timeout=25  writecount=2  readcount=0  sdapin=C9  sclpin=A8  waitwritetime=5  forcestop=off  inputtypearray=[3 3 3 3]  outputtypearray=[1 3]  confstr="[\"C\",\"9\",\"A\",\"8\",\"1\",\"1\",\"6\",\"0\",\"I2C_DutyCycle_2\",\"5\",\"off\"]"  sampletime=-1  sampletimestr=-1  blockid=CameraOV7670Init_WhileIterator_CommonConf_SubsystemI2CMasterReadWrite
  Register List : Subsystem  mask{register=uint8([122,123,124,125,126,127,128,129,130,131,132,133,134,135,136,137,19,21,0,16,13,20,165,171,36,37,38,159,160,161,166,167,168,169,170,19,14,15,22,30,33,34,41,51,53,55,56,57,60,77,78,105,116,141,142,143,144,145,146,150,154,176,177,178,179,184,67,68,69,70,71,72,89,90,91,92,93,94,100,101,102,148,149,108,109,110,111,106,1,2,19,21,79,80,81,82,83,84,85,86,87,88,65,63,117,118,76,119,75,201,65,86,52,59,164,150,157,158,9,59]), value=uint8([32,28,40,60,85,104,118,128,136,143,150,163,175,196,215,232,232,24,15,0,0,32,5,7,117,99,165,120,104,3,223,223,240,144,148,229,97,75,2,39,2,145,7,11,11,29,113,42,120,64,32,0,25,79,0,0,0,0,0,0,128,132,12,14,130,10,20,240,52,88,40,58,136,136,68,103,73,14,4,32,5,4,8,10,85,17,159,64,64,64,231,24,128,128,0,34,94,128,0,82,128,158,8,5,5,225,15,10,9,192,56,64,17,2,137,0,76,63,2,66])}
      mask prompts: register "Register Index"; value "Register Value"
      mask help:
      | Count:
      |  - Number of Register-Value pair.
      |  - Determine from lowest size, between Register and Value.
      | Reg:
      |  - Register index.
      | Value:
      |  - Data corresponding to specified register index.
  Relational Operator : RelationalOperator  Operator===  LogicOutDataTypeMode=boolean  LogicDataType=fixdt(0, 8)  OutDataTypeStr=boolean
  Slave Address : Constant  Value=slvaddr  OutDataTypeMode=uint8  OutDataType=fixdt(1, 16)  OutScaling=2^0  OutDataTypeStr=uint8
  Out1 : Outport
  wires:
  Slave Address/1 -> I2C Master Read/Write/1
  Data Store Read/1 -> Add/1, Register List/1(Index)
  I2C Master Read/Write/1 -> Compare To Zero/1
  Compare To Zero/1 -> Add/2
  Add/1 -> Relational Operator/2, Data Store Write/1
  Relational Operator/1 -> Out1/1
  Register List/2(Reg) -> I2C Master Read/Write/2
  Register List/3(Value) -> I2C Master Read/Write/3
  Register List/1(Count) -> Relational Operator/1

== system target_cam_robot_demo/Camera OV7670/Init_/While Iterator_/Picture Size_/Subsystem ==
  Enable : EnablePort
  Add : Sum  OutDataType=fixdt(1, 16)  OutScaling=2^-10
  Compare To Zero : simulink/Logic and Bit Operations/Compare To Zero  SystemSampleTime=-1  relop===  LogicOutDataTypeMode=uint8  ZeroCross=off
  Data Store Memory : DataStoreMemory  DataStoreName=Index  ReadBeforeWriteMsg=warning  WriteAfterWriteMsg=warning  WriteAfterReadMsg=warning  DataType=uint8  OutDataType=fixdt(1, 16)  OutScaling=2^0  OutDataTypeStr=uint8
  Data Store Read : DataStoreRead  DataStoreName=Index  SampleTime=-1
  Data Store Write : DataStoreWrite  DataStoreName=Index  SampleTime=-1
  I2C Master Read/Write : stm32f4_i2c_lib/I2C Master Read//Write  configuration=Transaction  module=1  lastmodule=3  transfer=Blocking  dutycycle=TLow/THigh = 2  clkspeed=400  timeout=25  writecount=2  readcount=0  sdapin=C9  sclpin=A8  waitwritetime=5  forcestop=off  inputtypearray=[3 3 3 3]  outputtypearray=[1 3]  confstr="[\"C\",\"9\",\"A\",\"8\",\"1\",\"1\",\"6\",\"0\",\"I2C_DutyCycle_2\",\"5\",\"off\"]"  sampletime=-1  sampletimestr=-1  blockid=CameraOV7670Init_WhileIterator_PictureSize_SubsystemI2CMasterReadWrite
  Relational Operator : RelationalOperator  Operator===  LogicOutDataTypeMode=boolean  LogicDataType=fixdt(0, 8)  OutDataTypeStr=boolean
  Slave Address : Constant  Value=slvaddr  OutDataTypeMode=uint8  OutDataType=fixdt(1, 16)  OutScaling=2^0  OutDataTypeStr=uint8
  Subsystem : Subsystem
  Out1 : Outport
  wires:
  Subsystem/1(Count) -> Relational Operator/1
  Subsystem/2(Reg) -> I2C Master Read/Write/2
  Subsystem/3(Value) -> I2C Master Read/Write/3
  Relational Operator/1 -> Out1/1
  Add/1 -> Data Store Write/1, Relational Operator/2
  Compare To Zero/1 -> Add/2
  I2C Master Read/Write/1 -> Compare To Zero/1
  Data Store Read/1 -> Subsystem/1(Index), Add/1
  Slave Address/1 -> I2C Master Read/Write/1

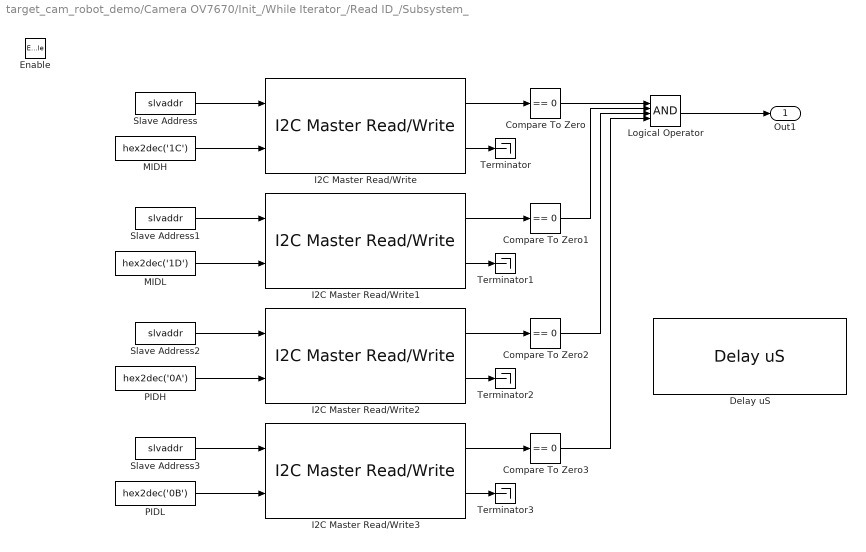
== system target_cam_robot_demo/Camera OV7670/Init_/While Iterator_/Read ID_/Subsystem_ ==
  Enable : EnablePort
  Compare To Zero{,1..3} (4 alike) : simulink/Logic and Bit Operations/Compare To Zero  SystemSampleTime=-1  relop===  LogicOutDataTypeMode=uint8  ZeroCross=off
  Delay uS : stm32f4_tim_lib/Delay uS  Priority=0  delaytime=300000  enableinput=off  enableoutput=off  inputtypearray=[0]  outputtypearray=[0]  sampletime=-1  sampletimestr=-1  blockid=CameraOV7670Init_WhileIterator_ReadID_Subsystem_DelayuS
  I2C Master Read/Write : stm32f4_i2c_lib/I2C Master Read//Write  configuration=Transaction  module=1  lastmodule=3  transfer=Blocking  dutycycle=TLow/THigh = 2  clkspeed=400  timeout=25  writecount=1  readcount=1  sdapin=C9  sclpin=A8  waitwritetime=0  forcestop=on  inputtypearray=[2 3 3]  outputtypearray=[2 3 3]  confstr="[\"C\",\"9\",\"A\",\"8\",\"1\",\"1\",\"6\",\"0\",\"I2C_DutyCycle_2\",\"0\",\"on\"]"  sampletime=-1  sampletimestr=-1  blockid=CameraOV7670Init_WhileIterator_ReadID_Subsystem_I2CMasterReadWrite
  I2C Master Read/Write1 : stm32f4_i2c_lib/I2C Master Read//Write  configuration=Transaction  module=1  lastmodule=3  transfer=Blocking  dutycycle=TLow/THigh = 2  clkspeed=400  timeout=25  writecount=1  readcount=1  sdapin=C9  sclpin=A8  waitwritetime=0  forcestop=on  inputtypearray=[2 3 3]  outputtypearray=[2 3 3]  confstr="[\"C\",\"9\",\"A\",\"8\",\"1\",\"1\",\"6\",\"0\",\"I2C_DutyCycle_2\",\"0\",\"on\"]"  sampletime=-1  sampletimestr=-1  blockid=CameraOV7670Init_WhileIterator_ReadID_Subsystem_I2CMasterReadWrite1
  I2C Master Read/Write2 : stm32f4_i2c_lib/I2C Master Read//Write  configuration=Transaction  module=1  lastmodule=3  transfer=Blocking  dutycycle=TLow/THigh = 2  clkspeed=400  timeout=25  writecount=1  readcount=1  sdapin=C9  sclpin=A8  waitwritetime=0  forcestop=on  inputtypearray=[2 3 3]  outputtypearray=[2 3 3]  confstr="[\"C\",\"9\",\"A\",\"8\",\"1\",\"1\",\"6\",\"0\",\"I2C_DutyCycle_2\",\"0\",\"on\"]"  sampletime=-1  sampletimestr=-1  blockid=CameraOV7670Init_WhileIterator_ReadID_Subsystem_I2CMasterReadWrite2
  I2C Master Read/Write3 : stm32f4_i2c_lib/I2C Master Read//Write  configuration=Transaction  module=1  lastmodule=3  transfer=Blocking  dutycycle=TLow/THigh = 2  clkspeed=400  timeout=25  writecount=1  readcount=1  sdapin=C9  sclpin=A8  waitwritetime=0  forcestop=on  inputtypearray=[2 3 3]  outputtypearray=[2 3 3]  confstr="[\"C\",\"9\",\"A\",\"8\",\"1\",\"1\",\"6\",\"0\",\"I2C_DutyCycle_2\",\"0\",\"on\"]"  sampletime=-1  sampletimestr=-1  blockid=CameraOV7670Init_WhileIterator_ReadID_Subsystem_I2CMasterReadWrite3
  Logical Operator : Logic  Inputs=4  AllPortsSameDT=off  OutDataTypeMode=boolean  LogicDataType=fixdt(0, 8)  OutDataTypeStr=boolean
  MIDH : Constant  Value=hex2dec('1C')  OutDataTypeMode=uint8  OutDataType=fixdt(1, 16)  OutScaling=2^0  OutDataTypeStr=uint8
  MIDL : Constant  Value=hex2dec('1D')  OutDataTypeMode=uint8  OutDataType=fixdt(1, 16)  OutScaling=2^0  OutDataTypeStr=uint8
  PIDH : Constant  Value=hex2dec('0A')  OutDataTypeMode=uint8  OutDataType=fixdt(1, 16)  OutScaling=2^0  OutDataTypeStr=uint8
  PIDL : Constant  Value=hex2dec('0B')  OutDataTypeMode=uint8  OutDataType=fixdt(1, 16)  OutScaling=2^0  OutDataTypeStr=uint8
  Slave Address{,1..3} (4 alike) : Constant  Value=slvaddr  OutDataTypeMode=uint8  OutDataType=fixdt(1, 16)  OutScaling=2^0  OutDataTypeStr=uint8
  Terminator{,1..3} (4 alike) : Terminator
  Out1 : Outport
  wires:
  I2C Master Read/Write3/2 -> Terminator3/1
  I2C Master Read/Write2/2 -> Terminator2/1
  I2C Master Read/Write1/2 -> Terminator1/1
  I2C Master Read/Write/2 -> Terminator/1
  Logical Operator/1 -> Out1/1
  Compare To Zero2/1 -> Logical Operator/3
  Compare To Zero3/1 -> Logical Operator/4
  Compare To Zero1/1 -> Logical Operator/2
  Compare To Zero/1 -> Logical Operator/1
  I2C Master Read/Write3/1 -> Compare To Zero3/1
  I2C Master Read/Write2/1 -> Compare To Zero2/1
  I2C Master Read/Write1/1 -> Compare To Zero1/1
  I2C Master Read/Write/1 -> Compare To Zero/1
  PIDL/1 -> I2C Master Read/Write3/2
  Slave Address3/1 -> I2C Master Read/Write3/1
  PIDH/1 -> I2C Master Read/Write2/2
  Slave Address2/1 -> I2C Master Read/Write2/1
  MIDL/1 -> I2C Master Read/Write1/2
  Slave Address1/1 -> I2C Master Read/Write1/1
  MIDH/1 -> I2C Master Read/Write/2
  Slave Address/1 -> I2C Master Read/Write/1

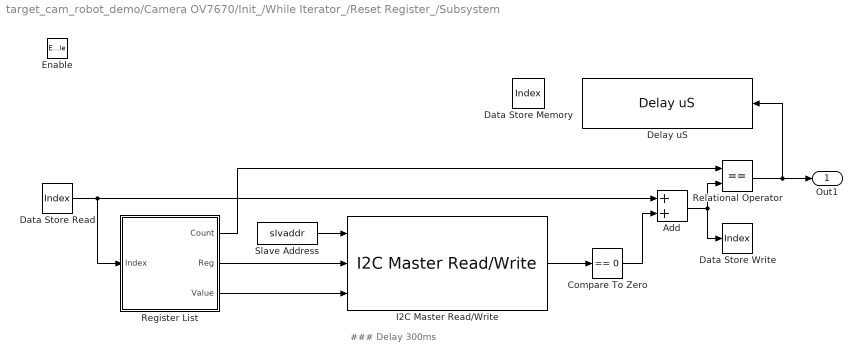
== system target_cam_robot_demo/Camera OV7670/Init_/While Iterator_/Reset Register_/Subsystem ==
  note: ### Delay 300ms
  Enable : EnablePort
  Add : Sum  OutDataType=fixdt(1, 16)  OutScaling=2^-10
  Compare To Zero : simulink/Logic and Bit Operations/Compare To Zero  SystemSampleTime=-1  relop===  LogicOutDataTypeMode=uint8  ZeroCross=off
  Data Store Memory : DataStoreMemory  DataStoreName=Index  ReadBeforeWriteMsg=warning  WriteAfterWriteMsg=warning  WriteAfterReadMsg=warning  DataType=uint8  OutDataType=fixdt(1, 16)  OutScaling=2^0  OutDataTypeStr=uint8
  Data Store Read : DataStoreRead  DataStoreName=Index  SampleTime=-1
  Data Store Write : DataStoreWrite  DataStoreName=Index  SampleTime=-1
  Delay uS : stm32f4_tim_lib/Delay uS  delaytime=200000  enableinput=on  enableoutput=off  inputtypearray=[1 -1]  outputtypearray=[0]  sampletime=-1  sampletimestr=-1  blockid=CameraOV7670Init_WhileIterator_ResetRegister_SubsystemDelayuS
  I2C Master Read/Write : stm32f4_i2c_lib/I2C Master Read//Write  configuration=Transaction  module=1  lastmodule=3  transfer=Blocking  dutycycle=TLow/THigh = 2  clkspeed=400  timeout=25  writecount=2  readcount=0  sdapin=C9  sclpin=A8  waitwritetime=300  forcestop=off  inputtypearray=[3 3 3 3]  outputtypearray=[1 3]  confstr="[\"C\",\"9\",\"A\",\"8\",\"1\",\"1\",\"6\",\"0\",\"I2C_DutyCycle_2\",\"300\",\"off\"]"  sampletime=-1  sampletimestr=-1  blockid=CameraOV7670Init_WhileIterator_ResetRegister_SubsystemI2CMasterReadWrite
  Register List : Subsystem  mask{register=uint8([hex2dec('12')]), value=uint8([hex2dec('80')])}
      mask prompts: register "Register Index"; value "Register Value"
      mask help:
      | Count:
      |  - Number of Register-Value pair.
      |  - Determine from lowest size, between Register and Value.
      | Reg:
      |  - Register index.
      | Value:
      |  - Data corresponding to specified register index.
  Relational Operator : RelationalOperator  Operator===  LogicOutDataTypeMode=boolean  LogicDataType=fixdt(0, 8)  OutDataTypeStr=boolean
  Slave Address : Constant  Value=slvaddr  OutDataTypeMode=uint8  OutDataType=fixdt(1, 16)  OutScaling=2^0  OutDataTypeStr=uint8
  Out1 : Outport
  wires:
  Slave Address/1 -> I2C Master Read/Write/1
  Data Store Read/1 -> Add/1, Register List/1(Index)
  I2C Master Read/Write/1 -> Compare To Zero/1
  Compare To Zero/1 -> Add/2
  Add/1 -> Relational Operator/2, Data Store Write/1
  Relational Operator/1 -> Delay uS/1, Out1/1
  Register List/2(Reg) -> I2C Master Read/Write/2
  Register List/3(Value) -> I2C Master Read/Write/3
  Register List/1(Count) -> Relational Operator/1

== system target_cam_robot_demo/Camera OV7670/Init_/While Iterator_/Clock Conf_/Subsystem/CLK24MHz_ ==
  Index : Inport  OutDataType=fixdt(1, 16)  OutScaling=2^0
  Enable : EnablePort
  Reg List_ : Subsystem  mask{register=uint8([17 107]), value=uint8([1 74])}
      mask prompts: register "Register Index"; value "Register Value"
      mask help:
      | Count:
      |  - Number of Register-Value pair.
      |  - Determine from lowest size, between Register and Value.
      | Reg:
      |  - Register index.
      | Value:
      |  - Data corresponding to specified register index.
  Count : Outport  OutDataType=fixdt(1, 16)  OutScaling=2^0
  Reg : Outport  Port=2  OutDataType=fixdt(1, 16)  OutScaling=2^0
  Value : Outport  Port=3  OutDataType=fixdt(1, 16)  OutScaling=2^0
  wires:
  Reg List_/1(Count) -> Count/1
  Reg List_/2(Reg) -> Reg/1
  Reg List_/3(Value) -> Value/1
  Index/1 -> Reg List_/1(Index)

== system target_cam_robot_demo/Camera OV7670/Init_/While Iterator_/Clock Conf_/Subsystem/CLK8MHz_ ==
  Index : Inport  OutDataType=fixdt(1, 16)  OutScaling=2^0
  Enable : EnablePort
  Reg List_ : Subsystem  mask{register=uint8([hex2dec('11') hex2dec('6B')]), value=uint8([hex2dec('00') hex2dec('80')])}
      mask prompts: register "Register Index"; value "Register Value"
      mask help:
      | Count:
      |  - Number of Register-Value pair.
      |  - Determine from lowest size, between Register and Value.
      | Reg:
      |  - Register index.
      | Value:
      |  - Data corresponding to specified register index.
  Count : Outport  OutDataType=fixdt(1, 16)  OutScaling=2^0
  Reg : Outport  Port=2  OutDataType=fixdt(1, 16)  OutScaling=2^0
  Value : Outport  Port=3  OutDataType=fixdt(1, 16)  OutScaling=2^0
  wires:
  Index/1 -> Reg List_/1(Index)
  Reg List_/3(Value) -> Value/1
  Reg List_/2(Reg) -> Reg/1
  Reg List_/1(Count) -> Count/1

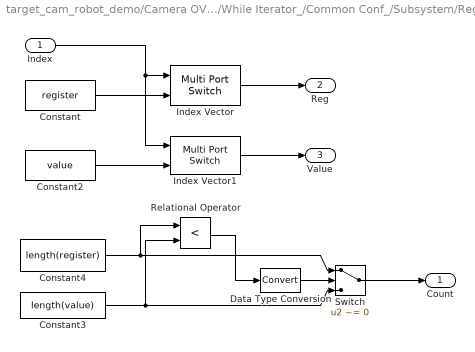
== system target_cam_robot_demo/Camera OV7670/Init_/While Iterator_/Common Conf_/Subsystem/Register List ==
  Index : Inport  OutDataType=fixdt(1, 16)  OutScaling=2^0
  Constant : Constant  Value=register  OutDataType=fixdt(1, 16)  OutScaling=2^0
  Constant2 : Constant  Value=value  OutDataType=fixdt(1, 16)  OutScaling=2^0
  Constant3 : Constant  Value=length(value)  OutDataType=fixdt(1, 16)  OutScaling=2^0
  Constant4 : Constant  Value=length(register)  OutDataType=fixdt(1, 16)  OutScaling=2^0
  Data Type Conversion : DataTypeConversion  OutDataType=fixdt(1, 16)  OutScaling=2^0
  Index Vector : MultiPortSwitch  Inputs=1  zeroidx=on  OutDataType=fixdt(1, 16)  OutScaling=2^0
  Index Vector1 : MultiPortSwitch  Inputs=1  zeroidx=on  OutDataType=fixdt(1, 16)  OutScaling=2^0
  Relational Operator : RelationalOperator  Operator=<  LogicOutDataTypeMode=boolean  LogicDataType=fixdt(0, 8)  OutDataTypeStr=boolean
  Switch : Switch  Criteria=u2 ~= 0  OutDataType=fixdt(1, 16)  OutScaling=2^0
  Count : Outport  OutDataType=fixdt(1, 16)  OutScaling=2^0
  Reg : Outport  Port=2  OutDataType=fixdt(1, 16)  OutScaling=2^0
  Value : Outport  Port=3  OutDataType=fixdt(1, 16)  OutScaling=2^0
  wires:
  Data Type Conversion/1 -> Switch/2
  Switch/1 -> Count/1
  Relational Operator/1 -> Data Type Conversion/1
  Constant3/1 -> Switch/3, Relational Operator/2
  Constant4/1 -> Switch/1, Relational Operator/1
  Index Vector1/1 -> Value/1
  Constant2/1 -> Index Vector1/2
  Index/1 -> Index Vector1/1, Index Vector/1
  Constant/1 -> Index Vector/2
  Index Vector/1 -> Reg/1
